simulink model "aula4"  (R2021a)
settings: Solver=VariableStepAuto  StartTime=0.0  StopTime=10.0  RelTol=1e-3
model workspace (MAT data in the model file):
  K1 = 1
  K2 = 1
  U0 = 1
settings Model: Creator=Lucas  LastModifiedBy=Lucas

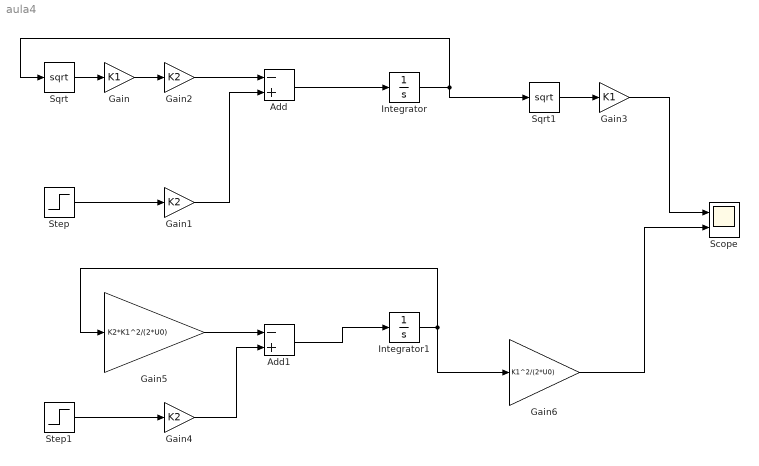
== system aula4 ==
  Add : Sum  Inputs=-+
  Add1 : Sum  Inputs=-+
  Gain : Gain  Gain=K1
  Gain1 : Gain  Gain=K2
  Gain2 : Gain  Gain=K2
  Gain3 : Gain  Gain=K1
  Gain4 : Gain  Gain=K2
  Gain5 : Gain  Gain=K2*K1^2/(2*U0)
  Gain6 : Gain  Gain=K1^2/(2*U0)
  Integrator : Integrator
  Integrator1 : Integrator
  Scope : Scope  NumInputPorts=2
  Sqrt : Sqrt  SaturateOnIntegerOverflow=on
  Sqrt1 : Sqrt  SaturateOnIntegerOverflow=on
  Step : Step  SampleTime=0
  Step1 : Step  SampleTime=0
  wires:
  Sqrt/1 -> Gain/1
  Step/1 -> Gain1/1
  Gain1/1 -> Add/2
  Gain/1 -> Gain2/1
  Add/1 -> Integrator/1
  Gain2/1 -> Add/1
  Integrator/1 -> Sqrt1/1, Sqrt/1
  Sqrt1/1 -> Gain3/1
  Gain3/1 -> Scope/1
  Step1/1 -> Gain4/1
  Gain4/1 -> Add1/2
  Gain5/1 -> Add1/1
  Add1/1 -> Integrator1/1
  Integrator1/1 -> Gain6/1, Gain5/1
  Gain6/1 -> Scope/2
